simulink subsystem "MyPieroModel"  (R2022b)
settings: Solver=VariableStepAuto  StartTime=0.0  StopTime=10.0  RelTol=1e-3
settings Model: Creator=Usuario  LastModifiedBy=Usuario
settings OptimizationCC: ReuseModelBlockBuffer=on
settings RTWCC: GPUComputeCapability=5.0

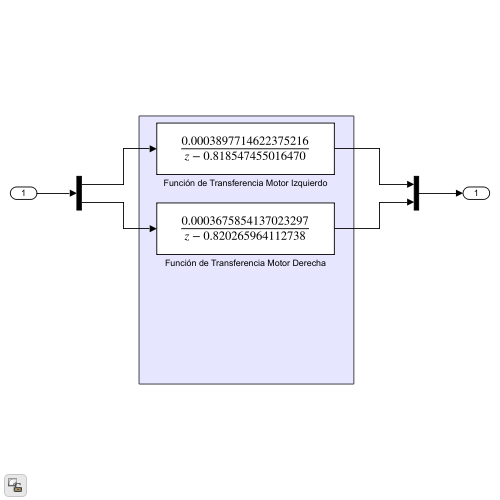
[thumbnail: Simulink's stored preview of the top-level diagram]
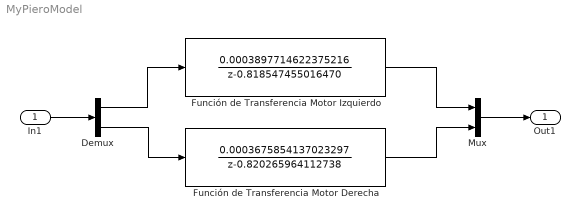
== system MyPieroModel ==
  In1 : Inport  OutDataTypeStr=double
  Demux : Demux  Outputs=2
  Función de Transferencia Motor Derecha : DiscreteTransferFcn  Numerator=0.0003675854137023297  Denominator=[1 -0.820265964112738]  SampleTime=0.01
  Función de Transferencia Motor Izquierdo : DiscreteTransferFcn  Numerator=0.0003897714622375216  Denominator=[1 -0.818547455016470]  SampleTime=0.01
  Mux : Mux  Inputs=2
  Out1 : Outport
  wires:
  Demux/2 -> Función de Transferencia Motor Derecha/1
  Demux/1 -> Función de Transferencia Motor Izquierdo/1
  Mux/1 -> Out1/1
  In1/1 -> Demux/1
  Función de Transferencia Motor Izquierdo/1 -> Mux/1
  Función de Transferencia Motor Derecha/1 -> Mux/2
